simulink model "statusLED"  (R2014b)
settings: Solver=FixedStepDiscrete  StartTime=0.0  StopTime=10.0  RelTol=1e-3
settings Model: Creator=Michael  LastModifiedBy=Michael
settings DataIOCC: SaveOutput=off  SaveTime=off
settings OptimizationCC: OptimizeModelRefInitCode=on  LifeSpan=1
settings HardwareCC: ProdBitPerChar=16  ProdBitPerInt=16  ProdBitPerPointer=16  ProdLargestAtomicInteger=Integer  ProdIntDivRoundTo=Zero  ProdEndianess=LittleEndian  ProdWordSize=16  ProdHWDeviceType=Texas Instruments->C2000
settings RTWCC: SystemTargetFile=idelink_ert.tlc  GenerateMakefile=off  TemplateMakefile=none  Description=IDE Link ERT  ProcessScript=idelink_ert_make_rtw_hook  Toolchain=Texas Instruments Code Composer Studio v5 (C2000)
settings CodeAppCC: IgnoreCustomStorageClasses=off
settings TargetHardwareResources: Description=Target Hardware Resources Component

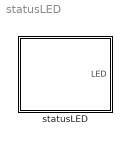
== system statusLED ==
  statusLED : Stateflow chart  TreatAsAtomicUnit=on

== stateflow chart statusLED/statusLED ==
  state statusLED
    state off
      entry: LED = false;
    state flash
      entry: LED = true;
    state on
      entry: LED = true;
    off -> on [order 2] : ON
    on -> off : OFF
    flash -> off : after(300,msec)
    off -> flash [order 1] : FLASH
  data: LED output boolean
  events: FLASH local FUNCTION_CALL_EVENT; ON local FUNCTION_CALL_EVENT; OFF local FUNCTION_CALL_EVENT
